simulink library "Pressure_Drop_changeD"  (Simulink 8.2)
settings: Solver=ode45  StartTime=0.0  StopTime=10.0  RelTol=1e-3
undefined symbols (not defined in the file): dia, DiameterLastPiece, DPConstant, DPLinear, DPQuadratic, Pressure
libraries: carnot x2, simulink x1
settings Model: Creator=drhf  LastModifiedBy=drhf

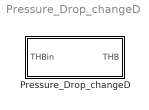
== system Pressure_Drop_changeD ==
  Pressure_Drop_changeD : Subsystem  mask(Pressure Drop Change Diameter){dia=dia}
      mask prompts: dia "Diameter in m"
      mask help: Calculates the pressure drop due to a diameter change at the inlet (of a pipe).
      mask Help: web(fullfile(path_carnot('help'),'Pressure_Drop_changeD.html'),'-helpbrowser')

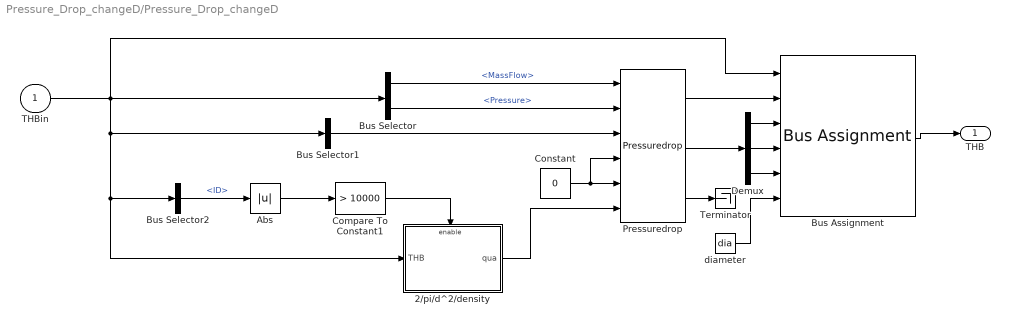
== system Pressure_Drop_changeD/Pressure_Drop_changeD ==
  THBin : Inport
  2/pi/d^2/density : Subsystem
  Abs : Abs
  Bus Assignment : BusAssignment  AssignedSignals=Pressure,DPConstant,DPLinear,DPQuadratic,DiameterLastPiece
  Bus Selector : BusSelector  OutputSignals=MassFlow,Pressure
  Bus Selector1 : BusSelector  OutputSignals=DPConstant,DPLinear,DPQuadratic  OutputAsBus=on
  Bus Selector2 : BusSelector  OutputSignals=ID
  Compare To Constant1 : simulink/Logic and Bit Operations/Compare To Constant  relop=>  const=10000  OutDataTypeStr=boolean
  Constant : Constant  Value=0
  Demux : Demux  Outputs=3
  Pressuredrop : carnot/Basic/Pressure_Drop/Pressuredrop
  Terminator : Terminator
  diameter : Constant  Value=dia
  THB : Outport
  wires:
  Pressuredrop/3 -> Terminator/1
  Compare To Constant1/1 -> 2/pi/d^2/density/Enable
  2/pi/d^2/density/1(qua) -> Pressuredrop/6
  Constant/1 -> Pressuredrop/4, Pressuredrop/5
  Bus Selector2/1 -> Abs/1  "<ID>"
  Bus Selector/2 -> Pressuredrop/2  "<Pressure>"
  Bus Selector/1 -> Pressuredrop/1  "<MassFlow>"
  Bus Selector1/1 -> Pressuredrop/3
  Abs/1 -> Compare To Constant1/1
  THBin/1 -> 2/pi/d^2/density/1(THB), Bus Selector2/1, Bus Selector1/1, Bus Selector/1, Bus Assignment/1
  Bus Assignment/1 -> THB/1
  Pressuredrop/1 -> Bus Assignment/2
  Demux/1 -> Bus Assignment/3
  Demux/2 -> Bus Assignment/4
  Demux/3 -> Bus Assignment/5
  Pressuredrop/2 -> Demux/1
  diameter/1 -> Bus Assignment/6

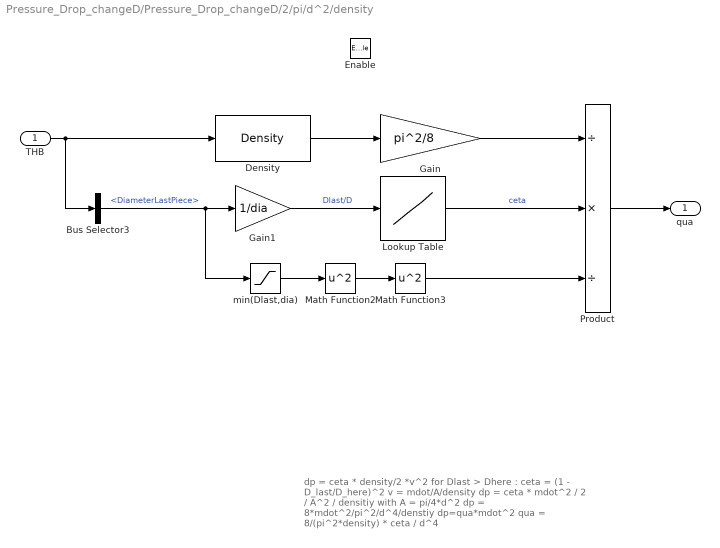
== system Pressure_Drop_changeD/Pressure_Drop_changeD/2/pi/d^2/density ==
  note: dp = ceta * density/2 *v^2
      | for Dlast > Dhere : ceta = (1 - D_last/D_here)^2
      | v = mdot/A/density
      | dp = ceta * mdot^2 / 2 / A^2 / densitiy
      | with A = pi/4*d^2
      | dp = 8*mdot^2/pi^2/d^4/denstiy
      | dp=qua*mdot^2
      | qua = 8/(pi^2*density) * ceta / d^4
  THB : Inport
  Enable : EnablePort
  Bus Selector3 : BusSelector  OutputSignals=DiameterLastPiece
  Density : carnot/Basic/Material_Properties/Density  VariantControl=CarlibClassic  INPUTARGUMENTS=THB  DEBUGLEVEL=DEBUGLEVEL  MAXTOTALWARNINGS=inf  MAXCONSECUTIVEWARNINGS=inf  WRITETOFILE=0  FILENAME='errors.txt'
  Gain : Gain  Gain=pi^2/8
  Gain1 : Gain  Gain=1/dia
  Lookup Table : Lookup  InputValues=[0:0.05:1, 10, 100]  Table="[(1 - [0:0.05:1]).^2,  1.2, 1.2]"
  Math Function2 : Math  Operator=square  SaturateOnIntegerOverflow=on
  Math Function3 : Math  Operator=square  SaturateOnIntegerOverflow=on
  Product : Product  Inputs=/*/  RndMeth=Zero
  min(Dlast,dia) : Saturate  UpperLimit=dia  LowerLimit=0
  qua : Outport
  wires:
  Lookup Table/1 -> Product/2  "ceta"
  Math Function3/1 -> Product/3
  Math Function2/1 -> Math Function3/1
  min(Dlast,dia)/1 -> Math Function2/1
  Gain1/1 -> Lookup Table/1  "Dlast/D"
  Product/1 -> qua/1
  Gain/1 -> Product/1
  Bus Selector3/1 -> min(Dlast,dia)/1, Gain1/1  "<DiameterLastPiece>"
  THB/1 -> Density/1, Bus Selector3/1
  Density/1 -> Gain/1
